simulink model "kinova_kinctrl1"  (R2020b)
settings: Solver=ode45  StartTime=0.0  StopTime=20.0  MaxStep=0.1  RelTol=1e-5  EnableMultiTasking=on
values from neighbouring files (symbols this model uses):
  K1 = K    (= 50)    [K_opt.m]    (also in kinova_mdl.m = Ks(1,switch_xd+1))
  switch_xd = 0    [kinova_mdl.m]
undefined symbols (not defined in the file or in its folder): qr
libraries: roblocks x4, simulink x1
settings Model: Creator=fernando  LastModifiedBy=lucas
settings DataIOCC: LimitDataPoints=on  SaveFormat=Array  SignalLoggingSaveFormat=ModelDataLogs  ReturnWorkspaceOutputs=off
settings OptimizationCC: ExpressionDepthLimit=2147483647  LifeSpan=inf
settings DebuggingCC: UnderspecifiedInitializationDetection=Classic  MergeDetectMultiDrivingBlocksExec=none  SolverPrmCheckMsg=warning  FcnCallInpInsideContextMsg=warning  AllowSymbolicDim=off  StateNameClashWarn=warning  SFUnexpectedBacktrackingDiag=warning  SFNoUnconditionalDefaultTransitionDiag=warning  SFExecutionAtInitializationDiag=none  ArithmeticOperatorsInVariantConditions=warning
settings HardwareCC: ProdBitPerPointer=32  ProdBitPerSizeT=32  ProdBitPerPtrDiffT=32  ProdLargestAtomicFloat=None  ProdIntDivRoundTo=Undefined  ProdEndianess=Unspecified  ProdWordSize=32  ProdHWDeviceType=32-bit Generic
settings ModelReferenceCC: PropagateSignalLabelsOutOfModel=off
settings SFSimCC: SimUseLocalCustomCode=off  CustomCodeUndefinedFunction=UseInterfaceOnly
settings RTWCC: RTWUseLocalCustomCode=off
settings CodeAppCC: StateflowObjectComments=on
settings GRTTargetCC: TargetLangStandard=C89/C90 (ANSI)  CombineOutputUpdateFcns=off  GRTInterface=on
settings ConfigComp: CovMetricSettings=dw  CovSaveCumulativeToWorkspaceVar=on  CovSaveSingleToWorkspaceVar=on  CovExternalEMLEnable=off

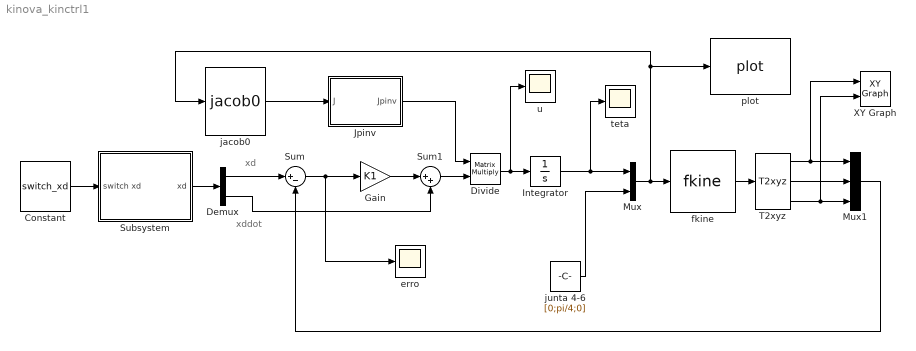
== system kinova_kinctrl1 ==
  note: xd
  note: xddot
  Constant : Constant  Value=switch_xd
  Demux : Demux  Outputs=2
  Divide : Product  Inputs=**  Multiplication=Matrix(*)
  Gain : Gain  Gain=K1
  Integrator : Integrator  InitialCondition=qr(1:4)
  Jpinv : MATLAB Function  TreatAsAtomicUnit=on
  Mux : Mux  Inputs=2
  Mux1 : Mux  Inputs=3
  Subsystem : Subsystem
  Sum : Sum  Inputs=|+-
  Sum1 : Sum  Inputs=|++
  T2xyz : roblocks/Toolbox/T2xyz
  XY Graph : simulink/Sinks/XY Graph  xmin=-0  xmax=0.8  ymin=-0.3  ymax=0.5  st=-1
  erro : Scope
  fkine : roblocks/Arm/fkine  robot=kinova
  "jacob0 " : roblocks/Arm/jacob0   robot=kinova
  junta 4-6 : Constant  Value=[0;pi/4;0]
  plot : roblocks/Arm/plot  robot=kinova  fps=5  holdplot=on
  teta : Scope
  u : Scope
  wires:
  Mux/1 -> fkine/1, plot/1, "jacob0 "/1
  Integrator/1 -> Mux/1, teta/1
  junta 4-6/1 -> Mux/2
  Divide/1 -> Integrator/1, u/1
  Jpinv/1(Jpinv) -> Divide/1
  Sum/1 -> Gain/1, erro/1
  fkine/1 -> T2xyz/1
  T2xyz/1 -> Mux1/1, XY Graph/1
  T2xyz/2 -> Mux1/2
  T2xyz/3 -> Mux1/3, XY Graph/2
  Mux1/1 -> Sum/2
  "jacob0 "/1 -> Jpinv/1(J)
  Demux/1 -> Sum/1
  Gain/1 -> Sum1/1
  Demux/2 -> Sum1/2
  Sum1/1 -> Divide/2
  Subsystem/1(xd) -> Demux/1
  Constant/1 -> Subsystem/1(switch xd)

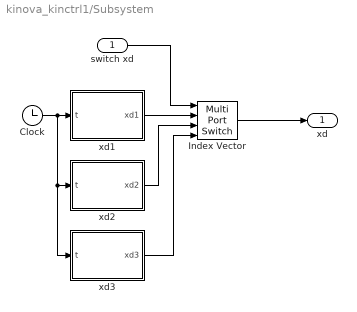
== system kinova_kinctrl1/Subsystem ==
  switch xd : Inport
  Clock : Clock
  Index Vector : MultiPortSwitch  DataPortOrder=Zero-based contiguous  zeroidx=on
  xd1 : MATLAB Function  TreatAsAtomicUnit=on
  xd2 : MATLAB Function  TreatAsAtomicUnit=on
  xd3 : MATLAB Function  TreatAsAtomicUnit=on
  xd : Outport
  wires:
  Clock/1 -> xd3/1(t), xd2/1(t), xd1/1(t)
  xd2/1(xd2) -> Index Vector/3
  xd1/1(xd1) -> Index Vector/2
  xd3/1(xd3) -> Index Vector/4
  Index Vector/1 -> xd/1
  switch xd/1 -> Index Vector/1

== matlab function kinova_kinctrl1/Subsystem/xd1 ==
  data: t input; xd1 output
function xd1  = fcn(t)
wn=2*pi/10;

xd= [0.456+0.075*cos(wn*t) 0 0.2+0.075*sin(wn*t)]';
xddot= [-0.075*wn*cos(wn*t) 0 0.075*wn*cos(wn*t)]';

xd1=[xd;xddot];

== matlab function kinova_kinctrl1/Subsystem/xd2 ==
  data: t input; xd2 output
function xd2  = fcn(t)
wn=2*pi/10;

xd= [0.456+0.075*cos(wn*t) 0.075*(sin(wn*t)+cos(wn*t)) 0.2+0.075*sin(wn*t)]';
xddot= [-0.075*wn*cos(wn*t) -0.075*wn*(cos(wn*t)+sin(wn*t)) 0.075*wn*cos(wn*t) ]';

xd2=[xd;xddot];

== matlab function kinova_kinctrl1/Subsystem/xd3 ==
  data: t input; xd3 output
function xd3  = fcn(t)
wn=2*pi/10;

xd= [0.456+0.075*(sin(4*wn*t)+sin(wn*t)) 0 0.2+0.075*(cos(wn*t)+cos(4*wn*t))]';
xddot= [0.075*wn*(cos(wn*t)+4*cos(4*wn*t)) 0 -0.075*wn*(sin(wn*t)+4*sin(wn*t))]';

xd3=[xd;xddot];

== matlab function kinova_kinctrl1/Jpinv ==
  data: J input; Jpinv output
function Jpinv = fcn(J)
%#codegen

Jpinv = pinv(J(1:3,1:4));
